simulink model "testes1"  (R2018b)
settings: Solver=FixedStepAuto  StartTime=0.0  StopTime=10  FixedStep=0.01  RelTol=1e-3
undefined symbols (not defined in the file or in its folder): DiscIntNeverNeededParam, teste3
libraries: simulink x2
settings Model: Creator=ubuntu  LastModifiedBy=ubuntu

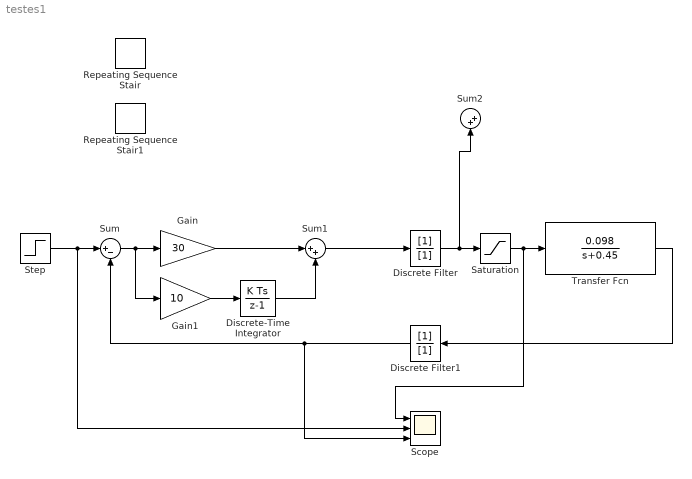
== system testes1 ==
  Discrete Filter : DiscreteFilter  Denominator=[1]  SampleTime=0.1
  Discrete Filter1 : DiscreteFilter  Denominator=[1]  SampleTime=0.1
  Discrete-Time Integrator : DiscreteIntegrator  SampleTime=0.1  ICPrevOutput=DiscIntNeverNeededParam  ICPrevScaledInput=DiscIntNeverNeededParam
  Gain : Gain  Gain=30
  Gain1 : Gain  Gain=10
  Repeating Sequence Stair : simulink/Sources/Repeating Sequence Stair  OutValues=teste3(:,3)  tsamp=0.1  OutMin=[]  OutMax=[]  OutDataTypeStr=double  OutputDataTypeScalingMode=double  OutDataType=fixdt(0,8)  ConRadixGroup=Best Precision: Vector-wise  OutScaling=2^-12
  Repeating Sequence Stair1 : simulink/Sources/Repeating Sequence Stair  OutValues=teste3(:,2)  tsamp=0.1  OutMin=[]  OutMax=[]  OutDataTypeStr=double  OutputDataTypeScalingMode=double  OutDataType=fixdt(0,8)  ConRadixGroup=Best Precision: Vector-wise  OutScaling=2^-12
  Saturation : Saturate  UpperLimit=24  LowerLimit=0
  Scope : Scope  NumInputPorts=3
  Step : Step  Time=5  Before=2.5  After=3  SampleTime=0
  Sum : Sum  Inputs=|+-
  Sum1 : Sum  Inputs=|++
  Sum2 : Sum  Inputs=|++
  Transfer Fcn : TransferFcn  Numerator=0.098  Denominator=[1 0.45]
  wires:
  Saturation/1 -> Scope/1, Transfer Fcn/1
  Step/1 -> Sum/1, Scope/2
  Sum/1 -> Gain1/1, Gain/1
  Transfer Fcn/1 -> Discrete Filter1/1
  Discrete Filter/1 -> Sum2/2, Saturation/1
  Discrete Filter1/1 -> Scope/3, Sum/2
  Gain/1 -> Sum1/1
  Gain1/1 -> Discrete-Time Integrator/1
  Discrete-Time Integrator/1 -> Sum1/2
  Sum1/1 -> Discrete Filter/1
